simulink model "ModifiedMotoHawkModel"  (R2016a)
settings: Solver=ode4  SolverMode=SingleTasking  StartTime=0.0  StopTime=10.0  FixedStep=0.001  RelTol=1e-3
values from neighbouring files (symbols this model uses):
  engineblendfactormap = [0 0 0 0 0 0 0 0 0 0 0 0 ... (420 elements, 21x20)]    [blendfactorvariables.mat]
  motorblendfactormap = [1 1 1 1 1 1 1 1 1 1 1 1 ... (420 elements, 21x20)]    [blendfactorvariables.mat]
  v = [0 5 10 15 20 25 30 35 40 45 50 55 ... (21 elements, 1x21)]    [blendfactorvariables.mat]
  x = [0 1 2 3 4 5 6 7 8 9 10 11 ... (20 elements, 1x20)]    [blendfactorvariables.mat]
undefined symbols (not defined in the file or in its folder): ECU565, motohawk_build_version, motohawk_trunc_name, motohawk_vardec_path
libraries: MotoHawk_lib x64
(part 2 of 2)

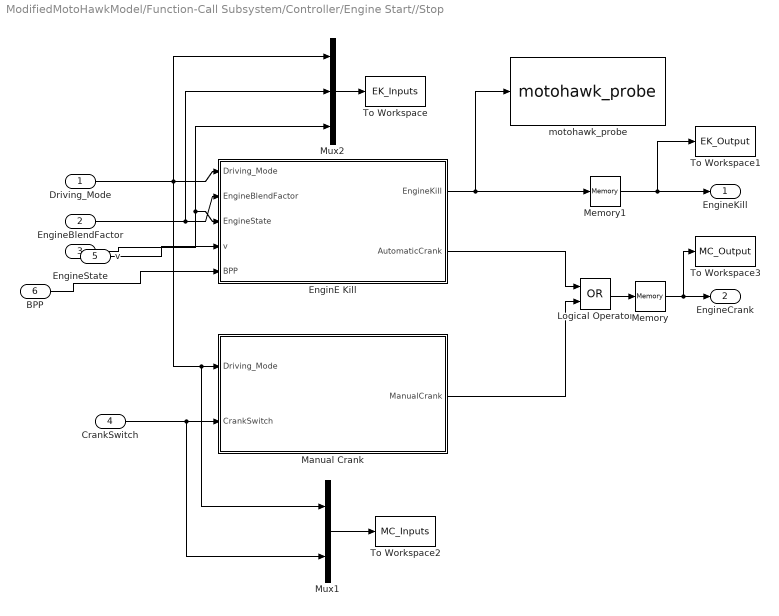
== system ModifiedMotoHawkModel/Function-Call Subsystem/Controller/Engine Start//Stop ==
  Driving_Mode : Inport
  EngineBlendFactor : Inport  Port=2
  EngineState : Inport  Port=3
  CrankSwitch : Inport  Port=4
  v : Inport  Port=5
  BPP : Inport  Port=6
  EnginE Kill : Stateflow chart  TreatAsAtomicUnit=on
  Logical Operator : Logic  Operator=OR  AllPortsSameDT=off  OutDataTypeStr=boolean
  Manual Crank : Stateflow chart  TreatAsAtomicUnit=on
  Memory : Memory  InheritSampleTime=on
  Memory1 : Memory  InheritSampleTime=on
  Mux1 : Mux  Inputs=2
  Mux2 : Mux  Inputs=3
  To Workspace : ToWorkspace  VariableName=EK_Inputs  SaveFormat=Structure With Time  SampleTime=-1
  To Workspace1 : ToWorkspace  VariableName=EK_Output  SaveFormat=Structure With Time  SampleTime=-1
  To Workspace2 : ToWorkspace  VariableName=MC_Inputs  SaveFormat=Structure With Time  SampleTime=-1
  To Workspace3 : ToWorkspace  VariableName=MC_Output  SaveFormat=Structure With Time  SampleTime=-1
  motohawk_probe : MotoHawk_lib/Calibration & Probing Blocks/motohawk_probe  nam='EngineKill'  show_more=off  name_source=Use Parameter  read_level=1  view_as=Number  enum_struct={'Disabled', 'Enabled'}  vector_style=Wide Row  use_help_units=off  help=''  units=''  use_header_enum=off  row_header_enum={}  col_header_enum={}  use_min_max=off  min_val=-inf  max_val=inf  use_precision=off  precision=''  gain=1  offset=0  exp=1  use_mototune_group=off  mototune_group=motohawk_vardec_path(gcb)
  EngineKill : Outport
  EngineCrank : Outport  Port=2
  wires:
  EnginE Kill/2(AutomaticCrank) -> Logical Operator/1
  CrankSwitch/1 -> Mux1/2, Manual Crank/2(CrankSwitch)
  EngineBlendFactor/1 -> Mux2/2, EnginE Kill/2(EngineBlendFactor)
  EngineState/1 -> EnginE Kill/3(EngineState), Mux2/3
  EnginE Kill/1(EngineKill) -> motohawk_probe/1, Memory1/1
  Driving_Mode/1 -> Mux2/1, Mux1/1, Manual Crank/1(Driving_Mode), EnginE Kill/1(Driving_Mode)
  Manual Crank/1(ManualCrank) -> Logical Operator/2
  Logical Operator/1 -> Memory/1
  Mux2/1 -> To Workspace/1
  Mux1/1 -> To Workspace2/1
  BPP/1 -> EnginE Kill/5(BPP)
  v/1 -> EnginE Kill/4(v)
  Memory/1 -> To Workspace3/1, EngineCrank/1
  Memory1/1 -> To Workspace1/1, EngineKill/1

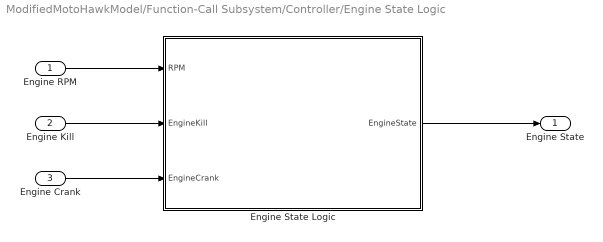
== system ModifiedMotoHawkModel/Function-Call Subsystem/Controller/Engine State Logic ==
  Engine RPM : Inport
  Engine Kill : Inport  Port=2
  Engine Crank : Inport  Port=3
  Engine State Logic : Stateflow chart  TreatAsAtomicUnit=on
  Engine State : Outport
  wires:
  Engine Kill/1 -> Engine State Logic/2(EngineKill)
  Engine RPM/1 -> Engine State Logic/1(RPM)
  Engine Crank/1 -> Engine State Logic/3(EngineCrank)
  Engine State Logic/1(EngineState) -> Engine State/1

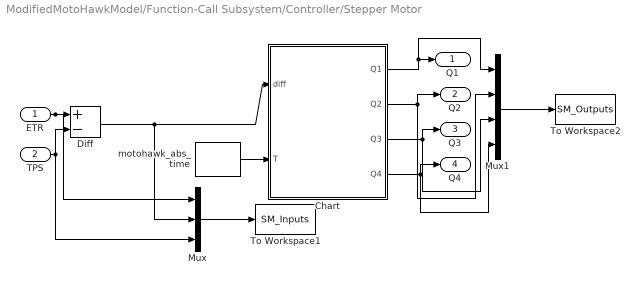
== system ModifiedMotoHawkModel/Function-Call Subsystem/Controller/Stepper Motor ==
  ETR : Inport
  TPS : Inport  Port=2
  Chart : Stateflow chart  TreatAsAtomicUnit=on
  Diff : Sum  Inputs=+-
  Mux : Mux  Inputs=3
  Mux1 : Mux
  To Workspace1 : ToWorkspace  VariableName=SM_Inputs  SaveFormat=Structure With Time  SampleTime=-1
  To Workspace2 : ToWorkspace  VariableName=SM_Outputs  SaveFormat=Structure With Time  SampleTime=-1
  motohawk_abs_time : MotoHawk_lib/Extra Development Blocks/motohawk_abs_time  mode=Seconds (double)  width=64 bit
  Q1 : Outport
  Q2 : Outport  Port=2
  Q3 : Outport  Port=3
  Q4 : Outport  Port=4
  wires:
  TPS/1 -> Mux/3, Diff/2
  Chart/2(Q2) -> Q2/1, Mux1/2
  Chart/3(Q3) -> Q3/1, Mux1/3
  Chart/4(Q4) -> Q4/1, Mux1/4
  Chart/1(Q1) -> Mux1/1, Q1/1
  ETR/1 -> Mux/1, Diff/1
  Diff/1 -> Mux/2, Chart/1(diff)
  Mux/1 -> To Workspace1/1
  Mux1/1 -> To Workspace2/1
  motohawk_abs_time/1 -> Chart/2(T)

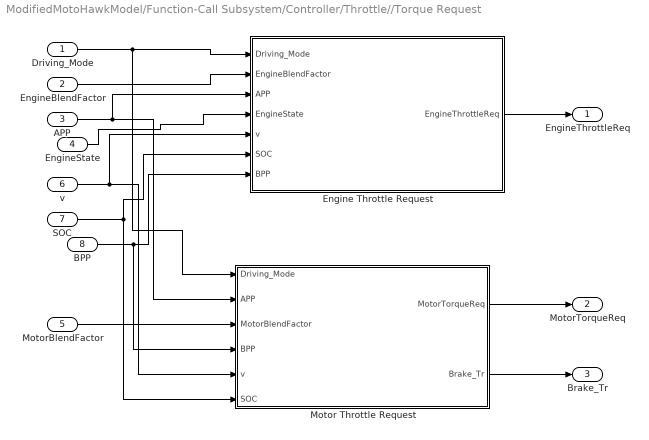
== system ModifiedMotoHawkModel/Function-Call Subsystem/Controller/Throttle//Torque Request ==
  Driving_Mode : Inport
  EngineBlendFactor : Inport  Port=2
  APP : Inport  Port=3
  EngineState : Inport  Port=4
  MotorBlendFactor : Inport  Port=5
  v : Inport  Port=6
  SOC : Inport  Port=7
  "BPP " : Inport  Port=8
  Engine Throttle Request : Stateflow chart  TreatAsAtomicUnit=on
  Motor Throttle Request : Stateflow chart  TreatAsAtomicUnit=on
  EngineThrottleReq : Outport
  MotorTorqueReq : Outport  Port=2
  Brake_Tr : Outport  Port=3
  wires:
  Driving_Mode/1 -> Motor Throttle Request/1(Driving_Mode), Engine Throttle Request/1(Driving_Mode)
  MotorBlendFactor/1 -> Motor Throttle Request/3(MotorBlendFactor)
  Motor Throttle Request/1(MotorTorqueReq) -> MotorTorqueReq/1
  APP/1 -> Engine Throttle Request/3(APP), Motor Throttle Request/2(APP)
  EngineBlendFactor/1 -> Engine Throttle Request/2(EngineBlendFactor)
  EngineState/1 -> Engine Throttle Request/4(EngineState)
  v/1 -> Motor Throttle Request/5(v), Engine Throttle Request/5(v)
  SOC/1 -> Engine Throttle Request/6(SOC), Motor Throttle Request/6(SOC)
  "BPP "/1 -> Motor Throttle Request/4(BPP), Engine Throttle Request/7(BPP)
  Motor Throttle Request/2(Brake_Tr) -> Brake_Tr/1
  Engine Throttle Request/1(EngineThrottleReq) -> EngineThrottleReq/1

== stateflow chart ModifiedMotoHawkModel/Function-Call Subsystem/Controller/Engine State Logic/Engine State Logic ==
  state EngineCrankState
    en,du:
    EngineState=2;
    EngineCrankTime=temporalCount(sec);
  state EngineOff
    en:EngineState=1;
  state EngineStartFail
    en:EngineState=5;
  state EngineOn
    en:EngineState=4;
  state EngineWarmup
    en,du:
    EngineState=3;
    EngineWarmUpTime=temporalCount(sec);
  (default) -> EngineOff
  EngineOff -> EngineCrankState : [EngineCrank==1 && EngineKill==0]
  EngineStartFail -> EngineOff
  EngineCrankState -> EngineStartFail [order 2] : [RPM<=800&&EngineCrankTime>1]
  EngineCrankState -> EngineWarmup [order 1] : [RPM>800&&EngineCrankTime>0.6]
  EngineOn -> EngineOff : [RPM<50 || EngineKill==1]
  EngineWarmup -> EngineStartFail [order 2] : [RPM<500 && EngineWarmUpTime>1]
  EngineWarmup -> EngineOn [order 1] : [RPM>=500 && EngineWarmUpTime>1]
  data: RPM input; EngineKill input; EngineCrank input; EngineState output; time local; EngineCrankTime local; EngineWarmUpTime local

== stateflow chart ModifiedMotoHawkModel/Function-Call Subsystem/Controller/Throttle//Torque Request/Engine Throttle Request ==
  state DWM
    state ElectricSolo
      en,du:EngineThrottleReq=0;
    state BlendingMode
      state EngineState23
        en,du:
        EngineThrottleReq=7.5;
      state OtherStates
        state ChargeSustain
          state Lowspeed
            en,du: EngineThrottleReq=APP*(1-EngineBlendFactor);
          state HighSpeed
            en,du:EngineThrottleReq=APP*EngineBlendFactor;
          HighSpeed -> Lowspeed : [v<10]
          Lowspeed -> HighSpeed : [v>=10]
          (default) -> HighSpeed
        state ChargeDepleting
          en,du:
          EngineThrottleReq=APP*EngineBlendFactor;
        ChargeDepleting -> ChargeSustain : [SOC<=0.3]
        ChargeSustain -> ChargeDepleting : [SOC>0.3]
        (default) -> ChargeDepleting
      OtherStates -> EngineState23 : [EngineState==2||EngineState==3]
      EngineState23 -> OtherStates : [EngineState~=2||EngineState~=3]
      (default) -> OtherStates
    state EngineSole
      en,du:EngineThrottleReq=APP;
    (junction 113) -> ElectricSolo [order 1] : [Driving_Mode==1]
    (junction 113) -> BlendingMode [order 2] : [Driving_Mode==2]
    BlendingMode -> (junction 113) : [Driving_Mode~=2]
    (junction 113) -> EngineSole [order 3] : [Driving_Mode==3]
    EngineSole -> (junction 113) : [Driving_Mode~=3]
    ElectricSolo -> (junction 113) : [Driving_Mode~=1]
    (default) -> ElectricSolo
  state Braking
    en,du: EngineThrottleReq=0;
  (default) -> DWM
  DWM -> Braking : [BPP>0]
  Braking -> DWM : [BPP<=0]
  data: Driving_Mode input; EngineBlendFactor input; APP input; EngineState input; EngineThrottleReq output; v input; SOC input; bat_protection_flag local; BPP input

== stateflow chart ModifiedMotoHawkModel/Function-Call Subsystem/Controller/Driving Mode/Driving Mode Controller ==
  state DM
    state EngineSolo
      du:Driving_Mode=3;
    state BlendingMode
      du:Driving_Mode=2;
    state ElectricSolo
      du:Driving_Mode=1;
    EngineSolo -> (junction 14) : [Engine_On_Switch==0||Motor_On_Switch==1]
    (junction 14) -> EngineSolo [order 1] : [Engine_On_Switch==1&&Motor_On_Switch==0&&v<1]
    (junction 14) -> ElectricSolo [order 3] : [Engine_On_Switch==0&&Motor_On_Switch==1&&v<1]
    BlendingMode -> (junction 14) : [Engine_On_Switch==1||Motor_On_Switch==1]
    (junction 14) -> BlendingMode [order 2] : [Engine_On_Switch==0&&Motor_On_Switch==0&&v<1]
    ElectricSolo -> (junction 14) : [Engine_On_Switch==1||Motor_On_Switch==0]
    (default) -> ElectricSolo
  state Nothing
  (default) -> Nothing
  Nothing -> DM : [v<=1]
  DM -> Nothing : [v>1]
  data: Engine_On_Switch input; Motor_On_Switch input; v input; Driving_Mode output

== stateflow chart ModifiedMotoHawkModel/Function-Call Subsystem/Controller/Throttle//Torque Request/Motor Throttle Request ==
  state NW
    state EngineSolo
      du:MotorTorqueReq=0;
    state ElectricSolo
      du:MotorTorqueReq=APP;
    state BlendingMode
      state ChargeSustain
        state Lowspeed
          en,du: MotorTorqueReq=APP*(1-MotorBlendFactor);
        state HighSpeed
          en,du:MotorTorqueReq=APP*MotorBlendFactor;
        HighSpeed -> Lowspeed : [v<=10]
        Lowspeed -> HighSpeed : [v>10]
        (default) -> HighSpeed
      state ChargeDepleting
        en,du:
        MotorTorqueReq=APP*MotorBlendFactor;
      ChargeDepleting -> ChargeSustain : [SOC<=0.3]
      ChargeSustain -> ChargeDepleting : [SOC>0.3]
      (default) -> ChargeDepleting
    (junction 5) -> EngineSolo [order 3] : [Driving_Mode==3]
    (junction 5) -> ElectricSolo [order 1] : [Driving_Mode==1]
    EngineSolo -> (junction 5) : [Driving_Mode~=3]
    ElectricSolo -> (junction 5) : [Driving_Mode~=1]
    BlendingMode -> (junction 5) : [Driving_Mode~=2]
    (junction 5) -> BlendingMode [order 2] : [Driving_Mode==2]
    (default) -> ElectricSolo
  state Braking
    state FrictionBrake
      du:MotorTorqueReq=0;
      Brake_Tr=BPP;
    state RegenerativeBrake
      du:MotorTorqueReq=BPP*0.75;
      Brake_Tr=BPP*0.5;
    (default) -> FrictionBrake
    FrictionBrake -> RegenerativeBrake : [v>2]
    RegenerativeBrake -> FrictionBrake : [v<=2]
  (default) -> NW
  NW -> Braking : [BPP>0]
  Braking -> NW : [BPP<=0]
  data: Driving_Mode input; APP input; MotorBlendFactor input; MotorTorqueReq output; BPP input; v input; Brake_Tr output; bat_protection_flag local; SOC input

== stateflow chart ModifiedMotoHawkModel/Function-Call Subsystem/Controller/Engine Start//Stop/EnginE Kill ==
  state EK
    state EngineSolo
      du:EngineKill=0;AutomaticCrank=0;
    state BlendingMode
      state a
        du:EngineKill=0;
        state c
          du:AutomaticCrank=1;
        state c1
          du:AutomaticCrank=0;
        (default) -> c
        c1 -> c : [EngineState==1]
        c -> c1 : [EngineState~=1]
      state b
        du:EngineKill=1;AutomaticCrank=0;
      (junction 13) -> a [order 1] : [EngineBlendFactor>0.01]
      a -> (junction 13) : [EngineBlendFactor<=0.01]
      b -> (junction 13) : [EngineBlendFactor>0.01]
      (junction 13) -> b [order 2] : [EngineBlendFactor<=0.01]
      (default) -> a
    state ElectricSolo
      du:EngineKill=1;AutomaticCrank=0;
    (junction 3) -> EngineSolo [order 3] : [Driving_Mode==3]
    EngineSolo -> (junction 3) : [Driving_Mode~=3]
    (junction 3) -> ElectricSolo [order 1] : [Driving_Mode==1]
    (junction 3) -> BlendingMode [order 2] : [Driving_Mode==2]
    BlendingMode -> (junction 3) : [Driving_Mode~=2]
    ElectricSolo -> (junction 3) : [Driving_Mode~=1]
    (default) -> ElectricSolo
  state Braking
    en:EngineKill=1;
  (default) -> EK
  EK -> Braking : [BPP>0]
  Braking -> EK : [BPP<=0]
  data: Driving_Mode input; EngineBlendFactor input; EngineKill output; EngineState input; AutomaticCrank output; v input; bat_protection_flag local; BPP input

== stateflow chart ModifiedMotoHawkModel/Function-Call Subsystem/Controller/Engine Start//Stop/Manual Crank ==
  state ElectricSolo
    du:ManualCrank=0;
  state EngineSolo
    state On
      du:ManualCrank=1;
    state Off
      du:ManualCrank=0;
    (junction 14) -> On [order 1] : [CrankSwitch==1]
    (junction 14) -> Off [order 2] : [CrankSwitch==0]
    Off -> (junction 14) : [CrankSwitch~=0]
    On -> (junction 14) : [CrankSwitch~=1]
    (default) -> Off
  state BlendingMode
    du:ManualCrank=0;
  (junction 1) -> EngineSolo [order 3] : [Driving_Mode==3]
  (junction 1) -> ElectricSolo [order 1] : [Driving_Mode==1]
  BlendingMode -> (junction 1) : [Driving_Mode~=2]
  EngineSolo -> (junction 1) : [Driving_Mode~=3]
  ElectricSolo -> (junction 1) : [Driving_Mode~=1]
  (junction 1) -> BlendingMode [order 2] : [Driving_Mode==2]
  (default) -> ElectricSolo
  data: Driving_Mode input; CrankSwitch input; ManualCrank output

== stateflow chart ModifiedMotoHawkModel/Function-Call Subsystem/Controller/E-motor start//stop model/E-Motor Start//Stop ==
  state EM
    state BlendingMode
      state B2
        du:Motor_On=0;
        du:Forward_Signal=1;
        du:Reverse_Signal=0;
      state B1
        du:Motor_On=1;
        du:Forward_Signal=1;
        du:Reverse_Signal=0;
      (junction 11) -> B2 [order 2] : [MotorBlendFactor<=0.01]
      (junction 11) -> B1 [order 1] : [MotorBlendFactor>0.01]
      B1 -> (junction 11) : [MotorBlendFactor<=0.01]
      B2 -> (junction 11) : [MotorBlendFactor>0.01]
      (default) -> B2
    state ElectricSolo
      du:Motor_On=1;
      du:Forward_Signal=ForwardSwitch;
      du:Reverse_Signal=ReverseSwitch;
    state EngineSolo
      du:Motor_On=0;
      du:Forward_Signal=0;
      du:Reverse_Signal=0;
    (default) -> ElectricSolo
    (junction 5) -> BlendingMode [order 2] : [Driving_Mode==2]
    (junction 5) -> ElectricSolo [order 1] : [Driving_Mode==1]
    ElectricSolo -> (junction 5) : [Driving_Mode~=1]
    BlendingMode -> (junction 5) : [Driving_Mode~=2]
    (junction 5) -> EngineSolo [order 3] : [Driving_Mode==3]
    EngineSolo -> (junction 5) : [Driving_Mode~=3]
  state Braking
    state FrictionBrake
      du:Motor_On=0;
      Forward_Signal=1;
      Reverse_Signal=0;
    state RegenerativeBrake
      du:Motor_On=1;
      Forward_Signal=1;
      Reverse_Signal=0;
    (default) -> FrictionBrake
    FrictionBrake -> RegenerativeBrake : [v>2]
    RegenerativeBrake -> FrictionBrake : [v<=2]
  (default) -> EM
  EM -> Braking : [BPP>0]
  Braking -> EM : [BPP<=0]
  data: Driving_Mode input; MotorBlendFactor input; ForwardSwitch input; ReverseSwitch input; Motor_On output; Forward_Signal output; Reverse_Signal output; v input; bat_protection_flag local; BPP input; SOC input

== stateflow chart ModifiedMotoHawkModel/Function-Call Subsystem/Controller/Stepper Motor/Chart ==
  state Step3
    en:T3=T;
    du:Q1=1;
    Q2=0;
    Q3=0;
    Q4=1;
  state Step4
    en:T4=T;
    du:Q1=0;
    Q2=0;
    Q3=0;
    Q4=1;
  state Step2
    en:T2=T;
    du:Q1=1;
    Q2=0;
    Q3=0;
    Q4=0;
  state Step1
    en:T1=T;
    du:Q1=1;
    Q2=0;
    Q3=1;
    Q4=0;
  state Step5
    en:T5=T;
    du:Q1=0;
    Q2=1;
    Q3=0;
    Q4=1;
  state Step8
    en:T8=T;
    du:Q1=0;
    Q2=0;
    Q3=1;
    Q4=0;
  state Step7
    en:T7=T;
    du:Q1=0;
    Q2=1;
    Q3=1;
    Q4=0;
  state Step6
    en:T6=T;
    du:Q1=0;
    Q2=1;
    Q3=0;
    Q4=0;
  Step4 -> Step3 [order 2] : [diff<=-1&&(T-T4)>5]
  Step2 -> Step3 [order 1] : [diff>=1&&(T-T2)>5]
  Step3 -> Step4 [order 1] : [diff>=1&&(T-T3)>5]
  Step1 -> Step2 [order 1] : [diff>=1&&(T-T1)>5]
  Step5 -> Step4 [order 2] : [diff<=-1&&(T-T5)>5]
  Step3 -> Step2 [order 2] : [diff<=-1&&(T-T3)>5]
  Step4 -> Step5 [order 1] : [diff>=1&&(T-T4)>5]
  Step2 -> Step1 [order 2] : [diff<=-1&&(T-T2)>5]
  (default) -> Step1
  Step6 -> Step5 [order 2] : [diff<=-1&&(T-T6)>5]
  Step1 -> Step8 [order 2] : [diff<=-1&&(T-T1)>5]
  Step5 -> Step6 [order 1] : [diff>=1&&(T-T5)>5]
  Step8 -> Step1 [order 1] : [diff>=1&&(T-T8)>5]
  Step7 -> Step8 [order 1] : [diff>=1&&(T-T7)>5]
  Step8 -> Step7 [order 2] : [diff<=-1&&(T-T8)>5]
  Step6 -> Step7 [order 1] : [diff>=1&&(T-T6)>5]
  Step7 -> Step6 [order 2] : [diff<=-1&&(T-T7)>5]
  data: diff input; Q1 output; Q2 output; Q3 output; Q4 output; T3 local; T5 local; T8 local; T2 local; T6 local; T4 local; T7 local; T1 local; T input
